simulink model "Buck_DCM_Controller_Due"  (R2020a)
settings: Solver=FixedStepAuto  StartTime=0.0  StopTime=inf  FixedStep=T  RelTol=1e-3  EnableMultiTasking=on
undefined symbols (not defined in the file): Iumax, Ki_I, Ki_IL, Kp_I, Kp_IL, Kp_Uc, Kp_W, Kphi, T, Ubat
libraries: arduinolib x11, eeStairGenerator x1
settings Model: SILPILModeSetting=veronly  ExtModeTrigDuration=2  Creator=Nguyen Tung  LastModifiedBy=Nguyen Tung
settings OptimizationCC: StrengthReduction=on  PassReuseOutputArgsAs=Individual arguments  ZeroExternalMemoryAtStartup=off  ZeroInternalMemoryAtStartup=off  MaxStackSize=64  OptimizeBlockOrder=speed  OptimizationPriority=Speed  OptimizationCustomize=off  MultiThreadedLoops=on  EfficientTunableParamExpr=on
settings DebuggingCC: ParameterTunabilityLossMsg=error
settings HardwareCC: ProdBitPerPointer=32  ProdBitPerSizeT=32  ProdBitPerPtrDiffT=32  ProdLargestAtomicInteger=Long  ProdLargestAtomicFloat=Double  ProdWordSize=32  ProdHWDeviceType=ARM Compatible->ARM Cortex
settings SFSimCC: MATLABDynamicMemAlloc=off
settings RTWCC: SystemTargetFile=ert.tlc  HardwareBoard=Arduino Due  TLCOptions=-aInlineSetEventsForThisBaseRateFcn=TLC_FALSE -aSuppressMultiTaskScheduler=TLC_FALSE -aRateBasedStepFcn=1  TemplateMakefile=ert_default_tmf  GenerateReport=on  Toolchain=Arduino ARM  BuildConfiguration=Faster Runs
settings CodeAppCC: ForceParamTrailComments=on  IgnoreCustomStorageClasses=off  OperatorAnnotations=on  SimulinkDataObjDesc=on  SFDataObjDesc=on  InsertBlockDesc=on
settings ERTTargetCC: SupportContinuousTime=on  SupportVariableSizeSignals=on  ExtModeStaticAllocSize=20000

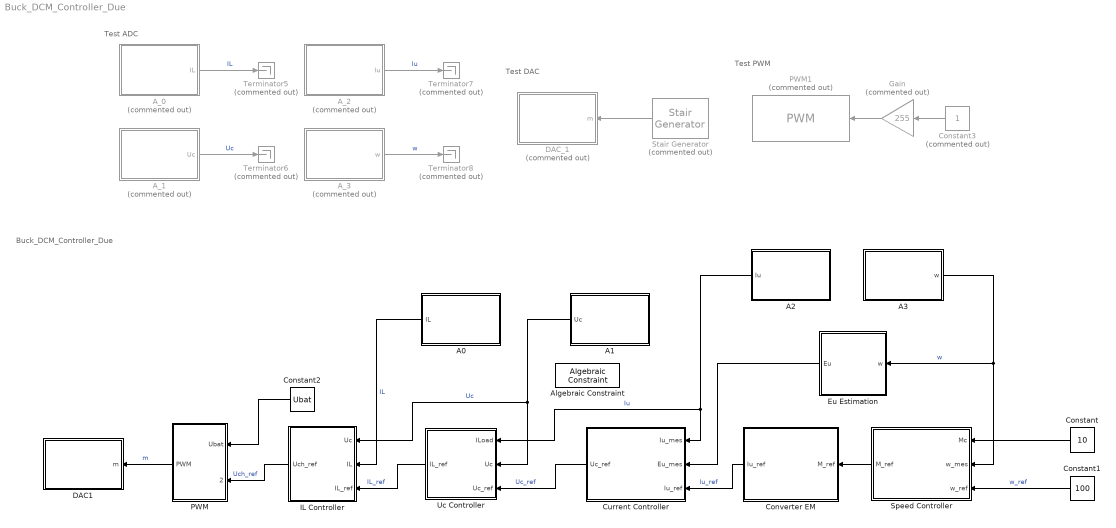
== system Buck_DCM_Controller_Due ==
  note: Buck_DCM_Controller_Due
  note: Test ADC
  note: Test PWM
  note: Test DAC
  A0 : Subsystem
  A1 : Subsystem
  A2 : Subsystem
  A3 : Subsystem
  A_0 : Subsystem  Commented=on
  A_1 : Subsystem  Commented=on
  A_2 : Subsystem  Commented=on
  A_3 : Subsystem  Commented=on
  Algebraic Constraint : AlgebraicConstraint
  Constant : Constant  Value=10
  Constant1 : Constant  Value=100
  Constant2 : Constant  Value=Ubat
  Constant3 : Constant  Commented=on
  Converter EM : Subsystem  AncestorBlock=simulink/SMC/Inversion EC avec mesure
      mask Display: plot(0,0,100,100,[10,30,90,70,10],[90,10,10,90,90])
  Current Controller : Subsystem  AncestorBlock=simulink/SMC/Asservissement Correcteur IP
      mask Display: plot(0,0,100,100, [10,30,90,70,10,90],[90,10,10,90,90,10])
  DAC1 : Subsystem
  DAC_1 : Subsystem  Commented=on
  Eu Estimation : Subsystem  AncestorBlock=simulink/REM/EC EM
      mask Display: plot(0,0,100,100, 1.4*[50,57.68,60.77,63.08,64.97,66.58,68,69.26,70.4, 	71.42,72.36,78.28,80,78.28,72.36,71.42,70.4, 	69.26,68,66.58,64.97,63.08,60.77,57.68,50,42.32, 	39.23,36.92,35.03,33.42,32,30.74,29.6,28.58, 	27.64,21.72,20,21.72,27.64,28.58,29.6,30.74,32, 	33.42,35.03,36.92,39.23,42.32,50]-20, 1.4*[20,21,22,23,24,25,26,27,28,29,30,40,50,60,70,71,72, 	73,74,75,76,77,78,79,80,79,78,77,76,75,74,73,72, 	71,70,60,50,40,30,29,28,27,26,25,24,23,22,21,20]-20)
  Gain : Gain  Commented=on  Gain=255
  IL Controller : Subsystem  AncestorBlock=simulink/SMC/Asservissement Correcteur IP
      mask Display: plot(0,0,100,100, [10,30,90,70,10,90],[90,10,10,90,90,10])
  PWM : Subsystem  AncestorBlock=simulink/SMC/Inversion EC avec mesure
      mask Display: plot(0,0,100,100,[10,30,90,70,10],[90,10,10,90,90])
  PWM1 : arduinolib/PWM  Commented=on  pinNumber=8  frequencyType=Specify  desiredFrequency=1000  achievableFrequency=1000
  Speed Controller : Subsystem  AncestorBlock=simulink/SMC/Asservissement Correcteur IP
      mask Display: plot(0,0,100,100, [10,30,90,70,10,90],[90,10,10,90,90,10])
  Stair Generator : eeStairGenerator/Stair Generator  Commented=on  LabelModeActiveChoice=Discrete  TimeInput=[0 2 4 6 8 10 12]  AmplitudeInput=[0 0.2 0.4 0.6 0.8 1 0]  SampleTime=T  RepeatPattern=on  OutDataTypeStr=double
      settings: SourceProductBaseCode=PS
  Terminator{5..8} (4 alike) : Terminator  Commented=on
  Uc Controller : Subsystem  AncestorBlock=simulink/SMC/Asservissement Correcteur IP
      mask Display: plot(0,0,100,100, [10,30,90,70,10,90],[90,10,10,90,90,10])
  wires:
  A_2/1(Iu) -> Terminator7/1  "Iu"
  A_0/1(IL) -> Terminator5/1  "IL"
  A_1/1(Uc) -> Terminator6/1  "Uc"
  A_3/1(w) -> Terminator8/1  "w"
  Uc Controller/1(IL_ref) -> IL Controller/3(IL_ref)  "IL_ref"
  Constant1/1 -> Speed Controller/3(w_ref)  "w_ref"
  Eu Estimation/1(Eu) -> Current Controller/2(Eu_mes)
  Current Controller/1(Uc_ref) -> Uc Controller/3(Uc_ref)  "Uc_ref"
  Converter EM/1(Iu_ref) -> Current Controller/3(Iu_ref)  "Iu_ref"
  Speed Controller/1(M_ref) -> Converter EM/1(M_ref)
  IL Controller/1(Uch_ref) -> PWM/2(Uch_ref)  "Uch_ref"
  A0/1(IL) -> IL Controller/2(IL)  "IL"
  A1/1(Uc) -> IL Controller/1(Uc), Uc Controller/2(Uc)  "Uc"
  A2/1(Iu) -> Uc Controller/1(ILoad), Current Controller/1(Iu_mes)  "Iu"
  A3/1(w) -> Speed Controller/2(w_mes), Eu Estimation/1(w)  "w"
  Constant/1 -> Speed Controller/1(Mc)
  Constant2/1 -> PWM/1(Ubat)
  Stair Generator/1 -> DAC_1/1(m)
  Constant3/1 -> Gain/1
  Gain/1 -> PWM1/1
  PWM/1(PWM) -> DAC1/1(m)  "m"

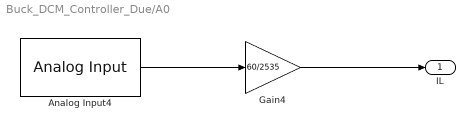
== system Buck_DCM_Controller_Due/A0 ==
  Analog Input4 : arduinolib/Analog Input  pinNumber=0  ReadResultsOnly=off  ConversionTriggerSource=Software  ExternalTriggerType=uint32( 0 )  OutputDataType=uint16  EnableConversionCompleteNotify=off  EnableOuputStatus=off  SampleTime=T  blockPlatform=arduino
  Gain4 : Gain  Gain=60/2535
  IL : Outport
  wires:
  Gain4/1 -> IL/1
  Analog Input4/1 -> Gain4/1

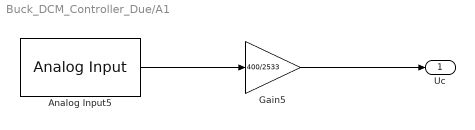
== system Buck_DCM_Controller_Due/A1 ==
  Analog Input5 : arduinolib/Analog Input  pinNumber=1  ReadResultsOnly=off  ConversionTriggerSource=Software  ExternalTriggerType=uint32( 0 )  OutputDataType=uint16  EnableConversionCompleteNotify=off  EnableOuputStatus=off  SampleTime=T  blockPlatform=arduino
  Gain5 : Gain  Gain=400/2533
  Uc : Outport
  wires:
  Analog Input5/1 -> Gain5/1
  Gain5/1 -> Uc/1

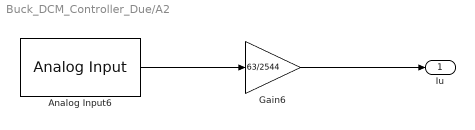
== system Buck_DCM_Controller_Due/A2 ==
  Analog Input6 : arduinolib/Analog Input  pinNumber=2  ReadResultsOnly=off  ConversionTriggerSource=Software  ExternalTriggerType=uint32( 0 )  OutputDataType=uint16  EnableConversionCompleteNotify=off  EnableOuputStatus=off  SampleTime=T  blockPlatform=arduino
  Gain6 : Gain  Gain=63/2544
  Iu : Outport
  wires:
  Analog Input6/1 -> Gain6/1
  Gain6/1 -> Iu/1

== system Buck_DCM_Controller_Due/A3 ==
  Analog Input7 : arduinolib/Analog Input  pinNumber=3  ReadResultsOnly=off  ConversionTriggerSource=Software  ExternalTriggerType=uint32( 0 )  OutputDataType=uint16  EnableConversionCompleteNotify=off  EnableOuputStatus=off  SampleTime=T  blockPlatform=arduino
  Gain7 : Gain  Gain=150/2545
  w : Outport
  wires:
  Analog Input7/1 -> Gain7/1
  Gain7/1 -> w/1

== system Buck_DCM_Controller_Due/A_0 ==
  Analog Input4 : arduinolib/Analog Input  pinNumber=0  ReadResultsOnly=off  ConversionTriggerSource=Software  ExternalTriggerType=uint32( 0 )  OutputDataType=uint16  EnableConversionCompleteNotify=off  EnableOuputStatus=off  SampleTime=T  blockPlatform=arduino
  Gain4 : Gain  Gain=60/2535
  IL : Outport
  wires:
  Analog Input4/1 -> Gain4/1
  Gain4/1 -> IL/1

== system Buck_DCM_Controller_Due/A_1 ==
  Analog Input5 : arduinolib/Analog Input  pinNumber=1  ReadResultsOnly=off  ConversionTriggerSource=Software  ExternalTriggerType=uint32( 0 )  OutputDataType=uint16  EnableConversionCompleteNotify=off  EnableOuputStatus=off  SampleTime=T  blockPlatform=arduino
  Gain5 : Gain  Gain=400/2533
  Uc : Outport
  wires:
  Analog Input5/1 -> Gain5/1
  Gain5/1 -> Uc/1

== system Buck_DCM_Controller_Due/A_2 ==
  Analog Input6 : arduinolib/Analog Input  pinNumber=2  ReadResultsOnly=off  ConversionTriggerSource=Software  ExternalTriggerType=uint32( 0 )  OutputDataType=uint16  EnableConversionCompleteNotify=off  EnableOuputStatus=off  SampleTime=T  blockPlatform=arduino
  Gain6 : Gain  Gain=63/2544
  Iu : Outport
  wires:
  Analog Input6/1 -> Gain6/1
  Gain6/1 -> Iu/1

== system Buck_DCM_Controller_Due/A_3 ==
  Analog Input7 : arduinolib/Analog Input  pinNumber=3  ReadResultsOnly=off  ConversionTriggerSource=Software  ExternalTriggerType=uint32( 0 )  OutputDataType=uint16  EnableConversionCompleteNotify=off  EnableOuputStatus=off  SampleTime=T  blockPlatform=arduino
  Gain7 : Gain  Gain=150/2545
  w : Outport
  wires:
  Analog Input7/1 -> Gain7/1
  Gain7/1 -> w/1

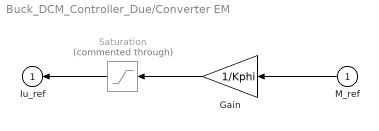
== system Buck_DCM_Controller_Due/Converter EM ==
  M_ref : Inport
  Gain : Gain  Gain=1/Kphi
  Saturation : Saturate  Commented=through  UpperLimit=Iumax  LowerLimit=0
  Iu_ref : Outport  InitialOutput=0  VectorParamsAs1DForOutWhenUnconnected=off
  wires:
  M_ref/1 -> Gain/1
  Gain/1 -> Saturation/1
  Saturation/1 -> Iu_ref/1

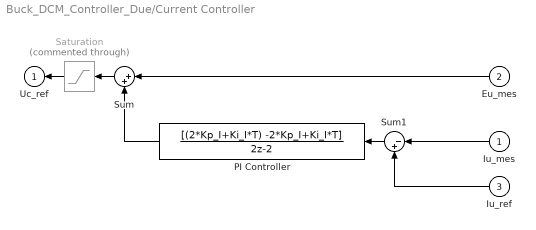
== system Buck_DCM_Controller_Due/Current Controller ==
  Iu_mes : Inport
  Eu_mes : Inport  Port=2
  Iu_ref : Inport  Port=3
  PI Controller : DiscreteTransferFcn  Numerator=[(2*Kp_I+Ki_I*T) -2*Kp_I+Ki_I*T]  Denominator=[2 -2]
  Saturation : Saturate  Commented=through  UpperLimit=Ubat  LowerLimit=0
  Sum : Sum  Inputs=|++
  Sum1 : Sum  Inputs=|-+
  Uc_ref : Outport  InitialOutput=0  VectorParamsAs1DForOutWhenUnconnected=off
  wires:
  Eu_mes/1 -> Sum/1
  Iu_mes/1 -> Sum1/1
  Sum1/1 -> PI Controller/1
  PI Controller/1 -> Sum/2
  Iu_ref/1 -> Sum1/2
  Sum/1 -> Saturation/1
  Saturation/1 -> Uc_ref/1

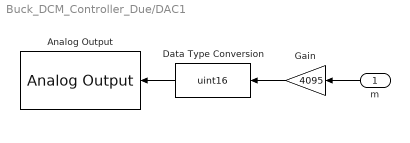
== system Buck_DCM_Controller_Due/DAC1 ==
  m : Inport
  Analog Output : arduinolib/Analog Output  DACpin=DAC1  blockPlatform=arduino
      settings: SourceProductBaseCode=ARDUINO
  Data Type Conversion : DataTypeConversion  OutDataTypeStr=uint16
  Gain : Gain  Gain=4095
  wires:
  m/1 -> Gain/1
  Gain/1 -> Data Type Conversion/1
  Data Type Conversion/1 -> Analog Output/1

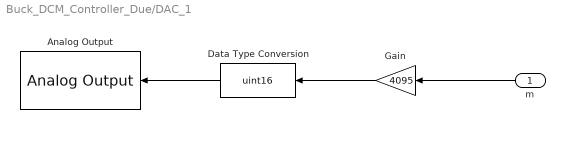
== system Buck_DCM_Controller_Due/DAC_1 ==
  m : Inport
  Analog Output : arduinolib/Analog Output  DACpin=DAC1  blockPlatform=arduino
      settings: SourceProductBaseCode=ARDUINO
  Data Type Conversion : DataTypeConversion  OutDataTypeStr=uint16
  Gain : Gain  Gain=4095
  wires:
  m/1 -> Gain/1
  Gain/1 -> Data Type Conversion/1
  Data Type Conversion/1 -> Analog Output/1

== system Buck_DCM_Controller_Due/Eu Estimation ==
  w : Inport
  Gain1 : Gain  Gain=Kphi
  Eu : Outport  InitialOutput=0  VectorParamsAs1DForOutWhenUnconnected=off
  wires:
  w/1 -> Gain1/1
  Gain1/1 -> Eu/1

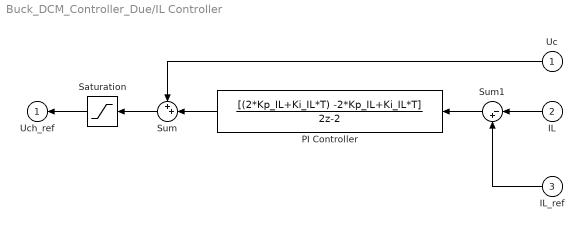
== system Buck_DCM_Controller_Due/IL Controller ==
  Uc : Inport
  IL : Inport  Port=2
  IL_ref : Inport  Port=3
  PI Controller : DiscreteTransferFcn  Numerator=[(2*Kp_IL+Ki_IL*T) -2*Kp_IL+Ki_IL*T]  Denominator=[2 -2]
  Saturation : Saturate  UpperLimit=Ubat  LowerLimit=0
  Sum : Sum  Inputs=++|
  Sum1 : Sum  Inputs=|-+
  Uch_ref : Outport  InitialOutput=0
  wires:
  Uc/1 -> Sum/1
  IL_ref/1 -> Sum1/2
  IL/1 -> Sum1/1
  Sum/1 -> Saturation/1
  PI Controller/1 -> Sum/2
  Sum1/1 -> PI Controller/1
  Saturation/1 -> Uch_ref/1

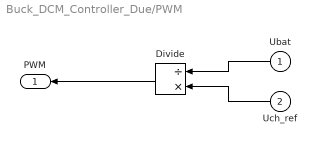
== system Buck_DCM_Controller_Due/PWM ==
  Ubat : Inport
  Uch_ref : Inport  Port=2
  Divide : Product  Inputs=/*
  PWM : Outport
  wires:
  Divide/1 -> PWM/1
  Ubat/1 -> Divide/1
  Uch_ref/1 -> Divide/2

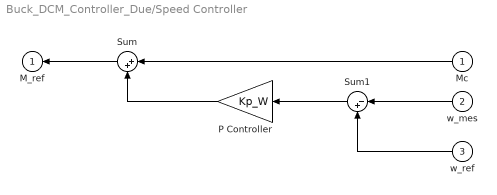
== system Buck_DCM_Controller_Due/Speed Controller ==
  Mc : Inport
  w_mes : Inport  Port=2
  w_ref : Inport  Port=3
  P Controller : Gain  Gain=Kp_W
  Sum : Sum  Inputs=|++
  Sum1 : Sum  Inputs=|-+
  M_ref : Outport  InitialOutput=0  VectorParamsAs1DForOutWhenUnconnected=off
  wires:
  Sum/1 -> M_ref/1
  w_ref/1 -> Sum1/2
  Sum1/1 -> P Controller/1
  P Controller/1 -> Sum/2
  Mc/1 -> Sum/1
  w_mes/1 -> Sum1/1

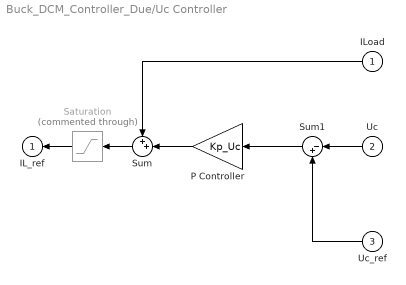
== system Buck_DCM_Controller_Due/Uc Controller ==
  ILoad : Inport
  Uc : Inport  Port=2
  Uc_ref : Inport  Port=3
  P Controller : Gain  Gain=Kp_Uc
  Saturation : Saturate  Commented=through  UpperLimit=Iumax  LowerLimit=0
  Sum : Sum  Inputs=++|
  Sum1 : Sum  Inputs=|-+
  IL_ref : Outport  InitialOutput=0
  wires:
  Uc/1 -> Sum1/1
  Uc_ref/1 -> Sum1/2
  Sum1/1 -> P Controller/1
  P Controller/1 -> Sum/2
  ILoad/1 -> Sum/1
  Sum/1 -> Saturation/1
  Saturation/1 -> IL_ref/1
